simulink library "BechamoNasaOpenModels"  (R2024a)
settings: Solver=VariableStepAuto  StartTime=0.0  StopTime=10.0  RelTol=1e-3
values from neighbouring files (symbols this model uses):
  Cl_aileron_wing_1 = Cl_mat.Claileron_wing.axes1.value    [setupMavrik.m]
  Cl_aileron_wing_2 = Cl_mat.Claileron_wing.axes2.value    [setupMavrik.m]
  Cl_aileron_wing_3 = Cl_mat.Claileron_wing.axes3.value    [setupMavrik.m]
  Cl_aileron_wing_val = Cl_mat.Claileron_wing.value    [setupMavrik.m]
  Cl_elevator_tail_1 = Cl_mat.Clelevator_tail.axes1.value    [setupMavrik.m]
  Cl_elevator_tail_2 = Cl_mat.Clelevator_tail.axes2.value    [setupMavrik.m]
  Cl_elevator_tail_3 = Cl_mat.Clelevator_tail.axes3.value    [setupMavrik.m]
  Cl_elevator_tail_val = Cl_mat.Clelevator_tail.value    [setupMavrik.m]
  Cl_flap_wing_1 = Cl_mat.Clflap_wing.axes1.value    [setupMavrik.m]
  Cl_flap_wing_2 = Cl_mat.Clflap_wing.axes2.value    [setupMavrik.m]
  Cl_flap_wing_3 = Cl_mat.Clflap_wing.axes3.value    [setupMavrik.m]
  Cl_flap_wing_val = Cl_mat.Clflap_wing.value    [setupMavrik.m]
  Cl_hover_fuse_1 = Cl_mat.Clhover_fuse.axes1.value    [setupMavrik.m]
  Cl_hover_fuse_2 = Cl_mat.Clhover_fuse.axes2.value    [setupMavrik.m]
  Cl_hover_fuse_3 = Cl_mat.Clhover_fuse.axes3.value    [setupMavrik.m]
  Cl_hover_fuse_val = Cl_mat.Clhover_fuse.value    [setupMavrik.m]
  Cl_rudder_tail_1 = Cl_mat.Clrudder_tail.axes1.value    [setupMavrik.m]
  Cl_rudder_tail_2 = Cl_mat.Clrudder_tail.axes2.value    [setupMavrik.m]
  Cl_rudder_tail_3 = Cl_mat.Clrudder_tail.axes3.value    [setupMavrik.m]
  Cl_rudder_tail_val = Cl_mat.Clrudder_tail.value    [setupMavrik.m]
  Cl_tail_1 = Cl_mat.Cltail.axes1.value    [setupMavrik.m]
  Cl_tail_2 = Cl_mat.Cltail.axes2.value    [setupMavrik.m]
  Cl_tail_3 = Cl_mat.Cltail.axes3.value    [setupMavrik.m]
  Cl_tail_damp_p_1 = Cl_mat.Cltail_damp_p.axes1.value    [setupMavrik.m]
  Cl_tail_damp_p_2 = Cl_mat.Cltail_damp_p.axes2.value    [setupMavrik.m]
  Cl_tail_damp_p_3 = Cl_mat.Cltail_damp_p.axes3.value    [setupMavrik.m]
  Cl_tail_damp_p_val = Cl_mat.Cltail_damp_p.value    [setupMavrik.m]
  Cl_tail_damp_q_1 = Cl_mat.Cltail_damp_q.axes1.value    [setupMavrik.m]
  Cl_tail_damp_q_2 = Cl_mat.Cltail_damp_q.axes2.value    [setupMavrik.m]
  Cl_tail_damp_q_3 = Cl_mat.Cltail_damp_q.axes3.value    [setupMavrik.m]
  Cl_tail_damp_q_val = Cl_mat.Cltail_damp_q.value    [setupMavrik.m]
  Cl_tail_damp_r_1 = Cl_mat.Cltail_damp_r.axes1.value    [setupMavrik.m]
  Cl_tail_damp_r_2 = Cl_mat.Cltail_damp_r.axes2.value    [setupMavrik.m]
  Cl_tail_damp_r_3 = Cl_mat.Cltail_damp_r.axes3.value    [setupMavrik.m]
  Cl_tail_damp_r_val = Cl_mat.Cltail_damp_r.value    [setupMavrik.m]
  Cl_tail_val = Cl_mat.Cltail.value    [setupMavrik.m]
  Cl_wing_1 = Cl_mat.Clwing.axes1.value    [setupMavrik.m]
  Cl_wing_2 = Cl_mat.Clwing.axes2.value    [setupMavrik.m]
  Cl_wing_3 = Cl_mat.Clwing.axes3.value    [setupMavrik.m]
  Cl_wing_damp_p_1 = Cl_mat.Clwing_damp_p.axes1.value    [setupMavrik.m]
  Cl_wing_damp_p_2 = Cl_mat.Clwing_damp_p.axes2.value    [setupMavrik.m]
  Cl_wing_damp_p_3 = Cl_mat.Clwing_damp_p.axes3.value    [setupMavrik.m]
  Cl_wing_damp_p_val = Cl_mat.Clwing_damp_p.value    [setupMavrik.m]
  Cl_wing_damp_q_1 = Cl_mat.Clwing_damp_q.axes1.value    [setupMavrik.m]
  Cl_wing_damp_q_2 = Cl_mat.Clwing_damp_q.axes2.value    [setupMavrik.m]
  Cl_wing_damp_q_3 = Cl_mat.Clwing_damp_q.axes3.value    [setupMavrik.m]
  Cl_wing_damp_q_val = Cl_mat.Clwing_damp_q.value    [setupMavrik.m]
  Cl_wing_damp_r_1 = Cl_mat.Clwing_damp_r.axes1.value    [setupMavrik.m]
  Cl_wing_damp_r_2 = Cl_mat.Clwing_damp_r.axes2.value    [setupMavrik.m]
  Cl_wing_damp_r_3 = Cl_mat.Clwing_damp_r.axes3.value    [setupMavrik.m]
  Cl_wing_damp_r_val = Cl_mat.Clwing_damp_r.value    [setupMavrik.m]
  Cl_wing_val = Cl_mat.Clwing.value    [setupMavrik.m]
  Cm_aileron_wing_1 = Cm_mat.Cmaileron_wing.axes1.value    [setupMavrik.m]
  Cm_aileron_wing_2 = Cm_mat.Cmaileron_wing.axes2.value    [setupMavrik.m]
  Cm_aileron_wing_3 = Cm_mat.Cmaileron_wing.axes3.value    [setupMavrik.m]
  Cm_aileron_wing_val = Cm_mat.Cmaileron_wing.value    [setupMavrik.m]
  Cm_elevator_tail_1 = Cm_mat.Cmelevator_tail.axes1.value    [setupMavrik.m]
  Cm_elevator_tail_2 = Cm_mat.Cmelevator_tail.axes2.value    [setupMavrik.m]
  Cm_elevator_tail_3 = Cm_mat.Cmelevator_tail.axes3.value    [setupMavrik.m]
  Cm_elevator_tail_val = Cm_mat.Cmelevator_tail.value    [setupMavrik.m]
  Cm_flap_wing_1 = Cm_mat.Cmflap_wing.axes1.value    [setupMavrik.m]
  Cm_flap_wing_2 = Cm_mat.Cmflap_wing.axes2.value    [setupMavrik.m]
  Cm_flap_wing_3 = Cm_mat.Cmflap_wing.axes3.value    [setupMavrik.m]
  Cm_flap_wing_val = Cm_mat.Cmflap_wing.value    [setupMavrik.m]
  Cm_hover_fuse_1 = Cm_mat.Cmhover_fuse.axes1.value    [setupMavrik.m]
  Cm_hover_fuse_2 = Cm_mat.Cmhover_fuse.axes2.value    [setupMavrik.m]
  Cm_hover_fuse_3 = Cm_mat.Cmhover_fuse.axes3.value    [setupMavrik.m]
  Cm_hover_fuse_val = Cm_mat.Cmhover_fuse.value    [setupMavrik.m]
  Cm_rudder_tail_1 = Cm_mat.Cmrudder_tail.axes1.value    [setupMavrik.m]
  Cm_rudder_tail_2 = Cm_mat.Cmrudder_tail.axes2.value    [setupMavrik.m]
  Cm_rudder_tail_3 = Cm_mat.Cmrudder_tail.axes3.value    [setupMavrik.m]
  Cm_rudder_tail_val = Cm_mat.Cmrudder_tail.value    [setupMavrik.m]
  Cm_tail_1 = Cm_mat.Cmtail.axes1.value    [setupMavrik.m]
  Cm_tail_2 = Cm_mat.Cmtail.axes2.value    [setupMavrik.m]
  Cm_tail_3 = Cm_mat.Cmtail.axes3.value    [setupMavrik.m]
  Cm_tail_damp_p_1 = Cm_mat.Cmtail_damp_p.axes1.value    [setupMavrik.m]
  Cm_tail_damp_p_2 = Cm_mat.Cmtail_damp_p.axes2.value    [setupMavrik.m]
  Cm_tail_damp_p_3 = Cm_mat.Cmtail_damp_p.axes3.value    [setupMavrik.m]
  Cm_tail_damp_p_val = Cm_mat.Cmtail_damp_p.value    [setupMavrik.m]
  Cm_tail_damp_q_1 = Cm_mat.Cmtail_damp_q.axes1.value    [setupMavrik.m]
  Cm_tail_damp_q_2 = Cm_mat.Cmtail_damp_q.axes2.value    [setupMavrik.m]
  Cm_tail_damp_q_3 = Cm_mat.Cmtail_damp_q.axes3.value    [setupMavrik.m]
  Cm_tail_damp_q_val = Cm_mat.Cmtail_damp_q.value    [setupMavrik.m]
  Cm_tail_damp_r_1 = Cm_mat.Cmtail_damp_r.axes1.value    [setupMavrik.m]
  Cm_tail_damp_r_2 = Cm_mat.Cmtail_damp_r.axes2.value    [setupMavrik.m]
  Cm_tail_damp_r_3 = Cm_mat.Cmtail_damp_r.axes3.value    [setupMavrik.m]
  Cm_tail_damp_r_val = Cm_mat.Cmtail_damp_r.value    [setupMavrik.m]
  Cm_tail_val = Cm_mat.Cmtail.value    [setupMavrik.m]
  Cm_wing_1 = Cm_mat.Cmwing.axes1.value    [setupMavrik.m]
  Cm_wing_2 = Cm_mat.Cmwing.axes2.value    [setupMavrik.m]
  Cm_wing_3 = Cm_mat.Cmwing.axes3.value    [setupMavrik.m]
  Cm_wing_damp_p_1 = Cm_mat.Cmwing_damp_p.axes1.value    [setupMavrik.m]
  Cm_wing_damp_p_2 = Cm_mat.Cmwing_damp_p.axes2.value    [setupMavrik.m]
  Cm_wing_damp_p_3 = Cm_mat.Cmwing_damp_p.axes3.value    [setupMavrik.m]
  Cm_wing_damp_p_val = Cm_mat.Cmwing_damp_p.value    [setupMavrik.m]
  Cm_wing_damp_q_1 = Cm_mat.Cmwing_damp_q.axes1.value    [setupMavrik.m]
  Cm_wing_damp_q_2 = Cm_mat.Cmwing_damp_q.axes2.value    [setupMavrik.m]
  Cm_wing_damp_q_3 = Cm_mat.Cmwing_damp_q.axes3.value    [setupMavrik.m]
  Cm_wing_damp_q_val = Cm_mat.Cmwing_damp_q.value    [setupMavrik.m]
  Cm_wing_damp_r_1 = Cm_mat.Cmwing_damp_r.axes1.value    [setupMavrik.m]
  Cm_wing_damp_r_2 = Cm_mat.Cmwing_damp_r.axes2.value    [setupMavrik.m]
  Cm_wing_damp_r_3 = Cm_mat.Cmwing_damp_r.axes3.value    [setupMavrik.m]
  Cm_wing_damp_r_val = Cm_mat.Cmwing_damp_r.value    [setupMavrik.m]
  Cm_wing_val = Cm_mat.Cmwing.value    [setupMavrik.m]
  Cn_aileron_wing_1 = Cn_mat.Cnaileron_wing.axes1.value    [setupMavrik.m]
  Cn_aileron_wing_2 = Cn_mat.Cnaileron_wing.axes2.value    [setupMavrik.m]
  Cn_aileron_wing_3 = Cn_mat.Cnaileron_wing.axes3.value    [setupMavrik.m]
  Cn_aileron_wing_val = Cn_mat.Cnaileron_wing.value    [setupMavrik.m]
  Cn_elevator_tail_1 = Cn_mat.Cnelevator_tail.axes1.value    [setupMavrik.m]
  Cn_elevator_tail_2 = Cn_mat.Cnelevator_tail.axes2.value    [setupMavrik.m]
  Cn_elevator_tail_3 = Cn_mat.Cnelevator_tail.axes3.value    [setupMavrik.m]
  Cn_elevator_tail_val = Cn_mat.Cnelevator_tail.value    [setupMavrik.m]
  Cn_flap_wing_1 = Cn_mat.Cnflap_wing.axes1.value    [setupMavrik.m]
  Cn_flap_wing_2 = Cn_mat.Cnflap_wing.axes2.value    [setupMavrik.m]
  Cn_flap_wing_3 = Cn_mat.Cnflap_wing.axes3.value    [setupMavrik.m]
  Cn_flap_wing_val = Cn_mat.Cnflap_wing.value    [setupMavrik.m]
  Cn_hover_fuse_1 = Cn_mat.Cnhover_fuse.axes1.value    [setupMavrik.m]
  Cn_hover_fuse_2 = Cn_mat.Cnhover_fuse.axes2.value    [setupMavrik.m]
  Cn_hover_fuse_3 = Cn_mat.Cnhover_fuse.axes3.value    [setupMavrik.m]
  Cn_hover_fuse_val = Cn_mat.Cnhover_fuse.value    [setupMavrik.m]
  ... (+318 more)
libraries: matrix_library x15, shared6dof x1, sharedtransform x1
(part 5 of 19)

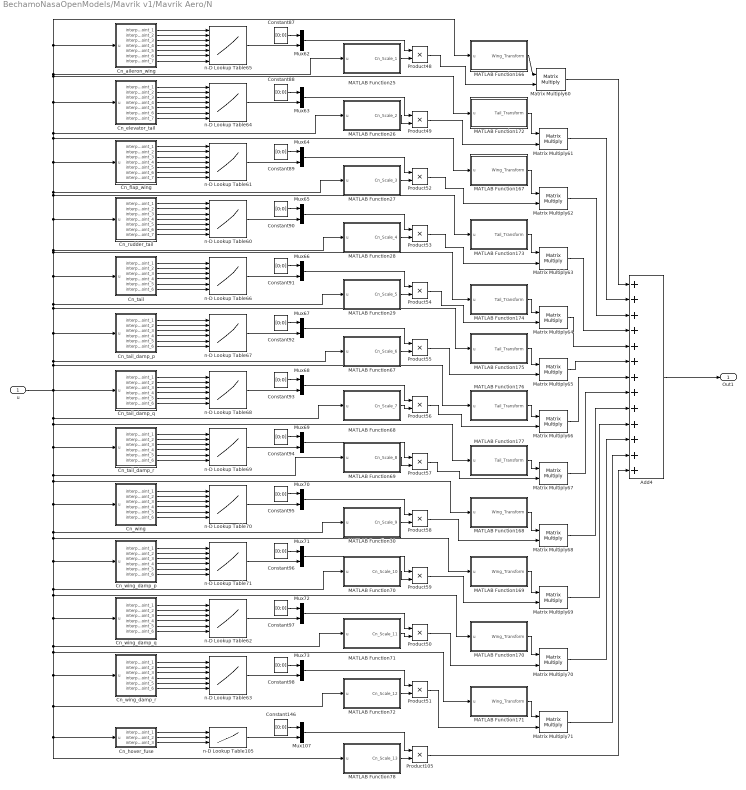
== system BechamoNasaOpenModels/Mavrik v1/Mavrik Aero/N ==
  u : Inport
  Add4 : Sum  Inputs=+++++++++++++
  Cn_aileron_wing : MATLAB Function  TreatAsAtomicUnit=on
  Cn_elevator_tail : MATLAB Function  TreatAsAtomicUnit=on
  Cn_flap_wing : MATLAB Function  TreatAsAtomicUnit=on
  Cn_hover_fuse : MATLAB Function  TreatAsAtomicUnit=on
  Cn_rudder_tail : MATLAB Function  TreatAsAtomicUnit=on
  Cn_tail : MATLAB Function  TreatAsAtomicUnit=on
  Cn_tail_damp_p : MATLAB Function  TreatAsAtomicUnit=on
  Cn_tail_damp_q : MATLAB Function  TreatAsAtomicUnit=on
  Cn_tail_damp_r : MATLAB Function  TreatAsAtomicUnit=on
  Cn_wing : MATLAB Function  TreatAsAtomicUnit=on
  Cn_wing_damp_p : MATLAB Function  TreatAsAtomicUnit=on
  Cn_wing_damp_q : MATLAB Function  TreatAsAtomicUnit=on
  Cn_wing_damp_r : MATLAB Function  TreatAsAtomicUnit=on
  Constant{87..98,146} (13 alike) : Constant  Value=[0;0]
  MATLAB Function166 : MATLAB Function  TreatAsAtomicUnit=on
  MATLAB Function167 : MATLAB Function  TreatAsAtomicUnit=on
  MATLAB Function168 : MATLAB Function  TreatAsAtomicUnit=on
  MATLAB Function169 : MATLAB Function  TreatAsAtomicUnit=on
  MATLAB Function170 : MATLAB Function  TreatAsAtomicUnit=on
  MATLAB Function171 : MATLAB Function  TreatAsAtomicUnit=on
  MATLAB Function172 : MATLAB Function  TreatAsAtomicUnit=on
  MATLAB Function173 : MATLAB Function  TreatAsAtomicUnit=on
  MATLAB Function174 : MATLAB Function  TreatAsAtomicUnit=on
  MATLAB Function175 : MATLAB Function  TreatAsAtomicUnit=on
  MATLAB Function176 : MATLAB Function  TreatAsAtomicUnit=on
  MATLAB Function177 : MATLAB Function  TreatAsAtomicUnit=on
  MATLAB Function25 : MATLAB Function  TreatAsAtomicUnit=on
  MATLAB Function26 : MATLAB Function  TreatAsAtomicUnit=on
  MATLAB Function27 : MATLAB Function  TreatAsAtomicUnit=on
  MATLAB Function28 : MATLAB Function  TreatAsAtomicUnit=on
  MATLAB Function29 : MATLAB Function  TreatAsAtomicUnit=on
  MATLAB Function30 : MATLAB Function  TreatAsAtomicUnit=on
  MATLAB Function67 : MATLAB Function  TreatAsAtomicUnit=on
  MATLAB Function68 : MATLAB Function  TreatAsAtomicUnit=on
  MATLAB Function69 : MATLAB Function  TreatAsAtomicUnit=on
  MATLAB Function70 : MATLAB Function  TreatAsAtomicUnit=on
  MATLAB Function71 : MATLAB Function  TreatAsAtomicUnit=on
  MATLAB Function72 : MATLAB Function  TreatAsAtomicUnit=on
  MATLAB Function78 : MATLAB Function  TreatAsAtomicUnit=on
  Matrix Multiply{60..71} (12 alike) : Product  Multiplication=Matrix(*)
  Mux{62..73,107} (13 alike) : Mux  Inputs=2
  Product{48..59,105} (13 alike) : Product
  n-D Lookup Table105 : Lookup_n-D  NumberOfTableDimensions=3  BreakpointsForDimension1=Cn_hover_fuse_1  BreakpointsForDimension2=Cn_hover_fuse_2  BreakpointsForDimension3=Cn_hover_fuse_3  BreakpointsForDimension4=CX_wing_damp_r_4  BreakpointsForDimension5=CX_wing_damp_r_5  BreakpointsForDimension6=CX_wing_damp_r_6  BreakpointsForDimension7=CX_flap_wing_7  Table=Cn_hover_fuse_val  InternalRulePriority=Speed  OutDataTypeStr=Inherit: Inherit via back propagation  RndMeth=Simplest
      settings: InputPortMap=u0,u1,u2
  n-D Lookup Table60 : Lookup_n-D  NumberOfTableDimensions=7  BreakpointsForDimension1=Cn_rudder_tail_1  BreakpointsForDimension2=Cn_rudder_tail_2  BreakpointsForDimension3=Cn_rudder_tail_3  BreakpointsForDimension4=Cn_rudder_tail_4  BreakpointsForDimension5=Cn_rudder_tail_5  BreakpointsForDimension6=Cn_rudder_tail_6  BreakpointsForDimension7=Cn_rudder_tail_7  Table=Cn_rudder_tail_val  InternalRulePriority=Speed  OutDataTypeStr=Inherit: Inherit via back propagation  RndMeth=Simplest
      settings: InputPortMap=u0,u1,u2,u3,u4,u5,u6
  n-D Lookup Table61 : Lookup_n-D  NumberOfTableDimensions=7  BreakpointsForDimension1=Cn_flap_wing_1  BreakpointsForDimension2=Cn_flap_wing_2  BreakpointsForDimension3=Cn_flap_wing_3  BreakpointsForDimension4=Cn_flap_wing_4  BreakpointsForDimension5=Cn_flap_wing_5  BreakpointsForDimension6=Cn_flap_wing_6  BreakpointsForDimension7=Cn_flap_wing_7  Table=Cn_flap_wing_val  InternalRulePriority=Speed  OutDataTypeStr=Inherit: Inherit via back propagation  RndMeth=Simplest
      settings: InputPortMap=u0,u1,u2,u3,u4,u5,u6
  n-D Lookup Table62 : Lookup_n-D  NumberOfTableDimensions=6  BreakpointsForDimension1=Cn_wing_damp_q_1  BreakpointsForDimension2=Cn_wing_damp_q_2  BreakpointsForDimension3=Cn_wing_damp_q_3  BreakpointsForDimension4=Cn_wing_damp_q_4  BreakpointsForDimension5=Cn_wing_damp_q_5  BreakpointsForDimension6=Cn_wing_damp_q_6  BreakpointsForDimension7=CX_flap_wing_7  Table=Cn_wing_damp_q_val  InternalRulePriority=Speed  OutDataTypeStr=Inherit: Inherit via back propagation  RndMeth=Simplest
      settings: InputPortMap=u0,u1,u2,u3,u4,u5
  n-D Lookup Table63 : Lookup_n-D  NumberOfTableDimensions=6  BreakpointsForDimension1=Cn_wing_damp_r_1  BreakpointsForDimension2=Cn_wing_damp_r_2  BreakpointsForDimension3=Cn_wing_damp_r_3  BreakpointsForDimension4=Cn_wing_damp_r_4  BreakpointsForDimension5=Cn_wing_damp_r_5  BreakpointsForDimension6=Cn_wing_damp_r_6  BreakpointsForDimension7=CX_flap_wing_7  Table=Cn_wing_damp_r_val  InternalRulePriority=Speed  OutDataTypeStr=Inherit: Inherit via back propagation  RndMeth=Simplest
      settings: InputPortMap=u0,u1,u2,u3,u4,u5
  n-D Lookup Table64 : Lookup_n-D  NumberOfTableDimensions=7  BreakpointsForDimension1=Cn_elevator_tail_1  BreakpointsForDimension2=Cn_elevator_tail_2  BreakpointsForDimension3=Cn_elevator_tail_3  BreakpointsForDimension4=Cn_elevator_tail_4  BreakpointsForDimension5=Cn_elevator_tail_5  BreakpointsForDimension6=Cn_elevator_tail_6  BreakpointsForDimension7=Cn_elevator_tail_7  Table=Cn_elevator_tail_val  InternalRulePriority=Speed  OutDataTypeStr=Inherit: Inherit via back propagation  RndMeth=Simplest
      settings: InputPortMap=u0,u1,u2,u3,u4,u5,u6
  n-D Lookup Table65 : Lookup_n-D  NumberOfTableDimensions=7  BreakpointsForDimension1=Cn_aileron_wing_1  BreakpointsForDimension2=Cn_aileron_wing_2  BreakpointsForDimension3=Cn_aileron_wing_3  BreakpointsForDimension4=Cn_aileron_wing_4  BreakpointsForDimension5=Cn_aileron_wing_5  BreakpointsForDimension6=Cn_aileron_wing_6  BreakpointsForDimension7=Cn_aileron_wing_7  Table=Cn_aileron_wing_val  InternalRulePriority=Speed  OutDataTypeStr=Inherit: Inherit via back propagation  RndMeth=Simplest
      settings: InputPortMap=u0,u1,u2,u3,u4,u5,u6
  n-D Lookup Table66 : Lookup_n-D  NumberOfTableDimensions=6  BreakpointsForDimension1=Cn_tail_1  BreakpointsForDimension2=Cn_tail_2  BreakpointsForDimension3=Cn_tail_3  BreakpointsForDimension4=Cn_tail_4  BreakpointsForDimension5=Cn_tail_5  BreakpointsForDimension6=Cn_tail_6  BreakpointsForDimension7=CX_tail_7  Table=Cn_tail_val  InternalRulePriority=Speed  OutDataTypeStr=Inherit: Inherit via back propagation  RndMeth=Simplest
      settings: InputPortMap=u0,u1,u2,u3,u4,u5
  n-D Lookup Table67 : Lookup_n-D  NumberOfTableDimensions=6  BreakpointsForDimension1=Cn_tail_damp_p_1  BreakpointsForDimension2=Cn_tail_damp_p_2  BreakpointsForDimension3=Cn_tail_damp_p_3  BreakpointsForDimension4=Cn_tail_damp_p_4  BreakpointsForDimension5=Cn_tail_damp_p_5  BreakpointsForDimension6=Cn_tail_damp_p_6  BreakpointsForDimension7=CX_tail_7  Table=Cn_tail_damp_p_val  InternalRulePriority=Speed  OutDataTypeStr=Inherit: Inherit via back propagation  RndMeth=Simplest
      settings: InputPortMap=u0,u1,u2,u3,u4,u5
  n-D Lookup Table68 : Lookup_n-D  NumberOfTableDimensions=6  BreakpointsForDimension1=Cn_tail_damp_q_1  BreakpointsForDimension2=Cn_tail_damp_q_2  BreakpointsForDimension3=Cn_tail_damp_q_3  BreakpointsForDimension4=Cn_tail_damp_q_4  BreakpointsForDimension5=Cn_tail_damp_q_5  BreakpointsForDimension6=Cn_tail_damp_q_6  BreakpointsForDimension7=CX_tail_7  Table=Cn_tail_damp_q_val  InternalRulePriority=Speed  OutDataTypeStr=Inherit: Inherit via back propagation  RndMeth=Simplest
      settings: InputPortMap=u0,u1,u2,u3,u4,u5
  n-D Lookup Table69 : Lookup_n-D  NumberOfTableDimensions=6  BreakpointsForDimension1=Cn_tail_damp_r_1  BreakpointsForDimension2=Cn_tail_damp_r_2  BreakpointsForDimension3=Cn_tail_damp_r_3  BreakpointsForDimension4=Cn_tail_damp_r_4  BreakpointsForDimension5=Cn_tail_damp_r_5  BreakpointsForDimension6=Cn_tail_damp_r_6  BreakpointsForDimension7=CX_tail_7  Table=Cn_tail_damp_r_val  InternalRulePriority=Speed  OutDataTypeStr=Inherit: Inherit via back propagation  RndMeth=Simplest
      settings: InputPortMap=u0,u1,u2,u3,u4,u5
  n-D Lookup Table70 : Lookup_n-D  NumberOfTableDimensions=6  BreakpointsForDimension1=Cn_wing_1  BreakpointsForDimension2=Cn_wing_2  BreakpointsForDimension3=Cn_wing_3  BreakpointsForDimension4=Cn_wing_4  BreakpointsForDimension5=Cn_wing_5  BreakpointsForDimension6=Cn_wing_6  BreakpointsForDimension7=CX_flap_wing_7  Table=Cn_wing_val  InternalRulePriority=Speed  OutDataTypeStr=Inherit: Inherit via back propagation  RndMeth=Simplest
      settings: InputPortMap=u0,u1,u2,u3,u4,u5
  n-D Lookup Table71 : Lookup_n-D  NumberOfTableDimensions=6  BreakpointsForDimension1=Cn_wing_damp_p_1  BreakpointsForDimension2=Cn_wing_damp_p_2  BreakpointsForDimension3=Cn_wing_damp_p_3  BreakpointsForDimension4=Cn_wing_damp_p_4  BreakpointsForDimension5=Cn_wing_damp_p_5  BreakpointsForDimension6=Cn_wing_damp_p_6  BreakpointsForDimension7=CX_flap_wing_7  Table=Cn_wing_damp_p_val  InternalRulePriority=Speed  OutDataTypeStr=Inherit: Inherit via back propagation  RndMeth=Simplest
      settings: InputPortMap=u0,u1,u2,u3,u4,u5
  Out1 : Outport
  wires:
  Cn_tail_damp_p/4(interp_point_4) -> n-D Lookup Table67/4
  Mux65/1 -> Product53/1
  n-D Lookup Table68/1 -> Mux68/2
  Product57/1 -> Matrix Multiply67/2
  n-D Lookup Table63/1 -> Mux73/2
  Constant96/1 -> Mux71/1
  n-D Lookup Table71/1 -> Mux71/2
  Matrix Multiply68/1 -> Add4/9
  Product54/1 -> Matrix Multiply64/2
  Matrix Multiply60/1 -> Add4/1
  Cn_flap_wing/7(interp_point_7) -> n-D Lookup Table61/7
  Cn_tail_damp_q/4(interp_point_4) -> n-D Lookup Table68/4
  Constant94/1 -> Mux69/1
  Cn_wing_damp_r/4(interp_point_4) -> n-D Lookup Table63/4
  Matrix Multiply61/1 -> Add4/2
  Cn_tail_damp_q/3(interp_point_3) -> n-D Lookup Table68/3
  Cn_tail_damp_p/5(interp_point_5) -> n-D Lookup Table67/5
  Mux62/1 -> Product48/1
  Cn_wing_damp_p/6(interp_point_6) -> n-D Lookup Table71/6
  Product48/1 -> Matrix Multiply60/2
  Mux66/1 -> Product54/1
  Cn_rudder_tail/7(interp_point_7) -> n-D Lookup Table60/7
  Cn_elevator_tail/5(interp_point_5) -> n-D Lookup Table64/5
  Constant92/1 -> Mux67/1
  Product52/1 -> Matrix Multiply62/2
  Cn_wing/1(interp_point_1) -> n-D Lookup Table70/1
  Cn_flap_wing/1(interp_point_1) -> n-D Lookup Table61/1
  Product50/1 -> Matrix Multiply70/2
  Matrix Multiply66/1 -> Add4/7
  Mux72/1 -> Product50/1
  Mux63/1 -> Product49/1
  n-D Lookup Table60/1 -> Mux65/2
  Mux71/1 -> Product59/1
  Mux68/1 -> Product56/1
  n-D Lookup Table65/1 -> Mux62/2
  Cn_tail/1(interp_point_1) -> n-D Lookup Table66/1
  Matrix Multiply70/1 -> Add4/11
  Cn_tail/4(interp_point_4) -> n-D Lookup Table66/4
  Mux64/1 -> Product52/1
  Matrix Multiply63/1 -> Add4/4
  MATLAB Function30/1(Cn_Scale_9) -> Product58/2
  Cn_aileron_wing/4(interp_point_4) -> n-D Lookup Table65/4
  Mux69/1 -> Product57/1
  n-D Lookup Table64/1 -> Mux63/2
  Cn_wing/6(interp_point_6) -> n-D Lookup Table70/6
  Constant88/1 -> Mux63/1
  Matrix Multiply67/1 -> Add4/8
  Product56/1 -> Matrix Multiply66/2
  Cn_tail_damp_p/6(interp_point_6) -> n-D Lookup Table67/6
  Constant91/1 -> Mux66/1
  MATLAB Function70/1(Cn_Scale_10) -> Product59/2
  Constant89/1 -> Mux64/1
  Cn_tail_damp_p/2(interp_point_2) -> n-D Lookup Table67/2
  Constant95/1 -> Mux70/1
  Cn_aileron_wing/2(interp_point_2) -> n-D Lookup Table65/2
  MATLAB Function26/1(Cn_Scale_2) -> Product49/2
  Cn_tail_damp_r/4(interp_point_4) -> n-D Lookup Table69/4
  MATLAB Function173/1(Tail_Transform) -> Matrix Multiply63/1
  Matrix Multiply69/1 -> Add4/10
  Cn_flap_wing/3(interp_point_3) -> n-D Lookup Table61/3
  MATLAB Function28/1(Cn_Scale_4) -> Product53/2
  MATLAB Function67/1(Cn_Scale_6) -> Product55/2
  Cn_tail_damp_q/2(interp_point_2) -> n-D Lookup Table68/2
  Cn_wing/5(interp_point_5) -> n-D Lookup Table70/5
  Product59/1 -> Matrix Multiply69/2
  Constant90/1 -> Mux65/1
  Cn_tail_damp_p/1(interp_point_1) -> n-D Lookup Table67/1
  MATLAB Function69/1(Cn_Scale_8) -> Product57/2
  MATLAB Function171/1(Wing_Transform) -> Matrix Multiply71/1
  Cn_elevator_tail/3(interp_point_3) -> n-D Lookup Table64/3
  Cn_hover_fuse/3(interp_point_3) -> n-D Lookup Table105/3
  Cn_flap_wing/6(interp_point_6) -> n-D Lookup Table61/6
  Cn_tail/2(interp_point_2) -> n-D Lookup Table66/2
  Cn_wing/4(interp_point_4) -> n-D Lookup Table70/4
  Product55/1 -> Matrix Multiply65/2
  Mux73/1 -> Product51/1
  Cn_hover_fuse/1(interp_point_1) -> n-D Lookup Table105/1
  Product105/1 -> Add4/13
  Mux107/1 -> Product105/1
  Cn_elevator_tail/1(interp_point_1) -> n-D Lookup Table64/1
  Cn_wing_damp_q/4(interp_point_4) -> n-D Lookup Table62/4
  Matrix Multiply62/1 -> Add4/3
  n-D Lookup Table61/1 -> Mux64/2
  Constant87/1 -> Mux62/1
  Constant97/1 -> Mux72/1
  Cn_wing_damp_p/4(interp_point_4) -> n-D Lookup Table71/4
  n-D Lookup Table69/1 -> Mux69/2
  Constant146/1 -> Mux107/1
  Cn_elevator_tail/4(interp_point_4) -> n-D Lookup Table64/4
  Product49/1 -> Matrix Multiply61/2
  Cn_wing_damp_r/6(interp_point_6) -> n-D Lookup Table63/6
  Cn_aileron_wing/5(interp_point_5) -> n-D Lookup Table65/5
  Product53/1 -> Matrix Multiply63/2
  Cn_aileron_wing/7(interp_point_7) -> n-D Lookup Table65/7
  Cn_tail/6(interp_point_6) -> n-D Lookup Table66/6
  MATLAB Function27/1(Cn_Scale_3) -> Product52/2
  MATLAB Function176/1(Tail_Transform) -> Matrix Multiply66/1
  MATLAB Function167/1(Wing_Transform) -> Matrix Multiply62/1
  Cn_rudder_tail/3(interp_point_3) -> n-D Lookup Table60/3
  Matrix Multiply71/1 -> Add4/12
  Cn_tail_damp_r/2(interp_point_2) -> n-D Lookup Table69/2
  Cn_tail/5(interp_point_5) -> n-D Lookup Table66/5
  Matrix Multiply64/1 -> Add4/5
  Cn_tail_damp_q/1(interp_point_1) -> n-D Lookup Table68/1
  Cn_tail_damp_p/3(interp_point_3) -> n-D Lookup Table67/3
  Cn_flap_wing/2(interp_point_2) -> n-D Lookup Table61/2
  Cn_wing_damp_q/6(interp_point_6) -> n-D Lookup Table62/6
  MATLAB Function25/1(Cn_Scale_1) -> Product48/2
  n-D Lookup Table70/1 -> Mux70/2
  Cn_rudder_tail/1(interp_point_1) -> n-D Lookup Table60/1
  Cn_tail_damp_q/5(interp_point_5) -> n-D Lookup Table68/5
  Constant93/1 -> Mux68/1
  n-D Lookup Table67/1 -> Mux67/2
  MATLAB Function175/1(Tail_Transform) -> Matrix Multiply65/1
  Cn_flap_wing/5(interp_point_5) -> n-D Lookup Table61/5
  Cn_flap_wing/4(interp_point_4) -> n-D Lookup Table61/4
  Cn_rudder_tail/5(interp_point_5) -> n-D Lookup Table60/5
  Cn_wing_damp_p/3(interp_point_3) -> n-D Lookup Table71/3
  Cn_elevator_tail/2(interp_point_2) -> n-D Lookup Table64/2
  Cn_tail_damp_q/6(interp_point_6) -> n-D Lookup Table68/6
  Cn_rudder_tail/4(interp_point_4) -> n-D Lookup Table60/4
  Cn_aileron_wing/6(interp_point_6) -> n-D Lookup Table65/6
  Cn_wing_damp_r/3(interp_point_3) -> n-D Lookup Table63/3
  MATLAB Function172/1(Tail_Transform) -> Matrix Multiply61/1
  Cn_wing_damp_r/5(interp_point_5) -> n-D Lookup Table63/5
  Cn_elevator_tail/7(interp_point_7) -> n-D Lookup Table64/7
  Cn_tail_damp_r/3(interp_point_3) -> n-D Lookup Table69/3
  Cn_tail_damp_r/6(interp_point_6) -> n-D Lookup Table69/6
  Cn_aileron_wing/1(interp_point_1) -> n-D Lookup Table65/1
  Cn_tail/3(interp_point_3) -> n-D Lookup Table66/3
  Cn_wing_damp_p/5(interp_point_5) -> n-D Lookup Table71/5
  Cn_wing_damp_p/2(interp_point_2) -> n-D Lookup Table71/2
  Cn_wing_damp_q/2(interp_point_2) -> n-D Lookup Table62/2
  Cn_wing_damp_r/2(interp_point_2) -> n-D Lookup Table63/2
  Cn_tail_damp_r/5(interp_point_5) -> n-D Lookup Table69/5
  Cn_wing/3(interp_point_3) -> n-D Lookup Table70/3
  MATLAB Function166/1(Wing_Transform) -> Matrix Multiply60/1
  Product51/1 -> Matrix Multiply71/2
  Cn_wing_damp_q/3(interp_point_3) -> n-D Lookup Table62/3
  n-D Lookup Table62/1 -> Mux72/2
  Add4/1 -> Out1/1
  Mux70/1 -> Product58/1
  Cn_wing_damp_q/5(interp_point_5) -> n-D Lookup Table62/5
  Mux67/1 -> Product55/1
  MATLAB Function168/1(Wing_Transform) -> Matrix Multiply68/1
  n-D Lookup Table66/1 -> Mux66/2
  Matrix Multiply65/1 -> Add4/6
  Constant98/1 -> Mux73/1
  MATLAB Function170/1(Wing_Transform) -> Matrix Multiply70/1
  MATLAB Function177/1(Tail_Transform) -> Matrix Multiply67/1
  MATLAB Function169/1(Wing_Transform) -> Matrix Multiply69/1
  Cn_elevator_tail/6(interp_point_6) -> n-D Lookup Table64/6
  MATLAB Function29/1(Cn_Scale_5) -> Product54/2
  Cn_aileron_wing/3(interp_point_3) -> n-D Lookup Table65/3
  MATLAB Function78/1(Cn_Scale_13) -> Product105/2
  Cn_wing/2(interp_point_2) -> n-D Lookup Table70/2
  Product58/1 -> Matrix Multiply68/2
  MATLAB Function68/1(Cn_Scale_7) -> Product56/2
  Cn_wing_damp_p/1(interp_point_1) -> n-D Lookup Table71/1
  MATLAB Function71/1(Cn_Scale_11) -> Product50/2
  Cn_wing_damp_q/1(interp_point_1) -> n-D Lookup Table62/1
  n-D Lookup Table105/1 -> Mux107/2
  Cn_rudder_tail/2(interp_point_2) -> n-D Lookup Table60/2
  Cn_wing_damp_r/1(interp_point_1) -> n-D Lookup Table63/1
  Cn_hover_fuse/2(interp_point_2) -> n-D Lookup Table105/2
  MATLAB Function174/1(Tail_Transform) -> Matrix Multiply64/1
  Cn_rudder_tail/6(interp_point_6) -> n-D Lookup Table60/6
  Cn_tail_damp_r/1(interp_point_1) -> n-D Lookup Table69/1
  MATLAB Function72/1(Cn_Scale_12) -> Product51/2
  u/1 -> MATLAB Function68/1(u), MATLAB Function69/1(u), MATLAB Function168/1(u), Cn_wing/1(u), MATLAB Function30/1(u), MATLAB Function169/1(u), Cn_wing_damp_p/1(u), MATLAB Function70/1(u), MATLAB Function170/1(u), Cn_wing_damp_q/1(u), MATLAB Function71/1(u), MATLAB Function171/1(u), Cn_wing_damp_r/1(u), MATLAB Function72/1(u), Cn_hover_fuse/1(u), MATLAB Function78/1(u), Cn_tail_damp_r/1(u), MATLAB Function177/1(u), MATLAB Function176/1(u), MATLAB Function67/1(u), Cn_tail_damp_p/1(u), MATLAB Function175/1(u), MATLAB Function29/1(u), Cn_tail/1(u), MATLAB Function174/1(u), MATLAB Function28/1(u), Cn_rudder_tail/1(u), MATLAB Function173/1(u), Cn_flap_wing/1(u), MATLAB Function167/1(u), MATLAB Function26/1(u), Cn_elevator_tail/1(u), Cn_aileron_wing/1(u), MATLAB Function166/1(u), MATLAB Function25/1(u), MATLAB Function172/1(u), MATLAB Function27/1(u), Cn_tail_damp_q/1(u)

== matlab function BechamoNasaOpenModels/Mavrik v1/Mavrik Aero/Ct/Ct_right_9 ==
  data: u input size=[1 45]; interp_point_1 output; interp_point_2 output; interp_point_3 output; interp_point_4 output
function [interp_point_1, interp_point_2, interp_point_3, interp_point_4] = fcn(u)

% Find Interpolation Points
variable_indices = struct('U', 1, 'alpha', 2, 'beta', 3, 'p', 4, 'q', 5, 'r', 6, 'wing_alpha', 7, 'wing_beta', 8, 'wing_RPM', 9, 'left_alpha', 10,...
    'right_alpha', 11, 'left_beta', 12, 'right_beta', 13, 'wing_prop_alpha', 14, 'wing_prop_beta', 15, 'tail_alpha', 16, 'tail_beta', 17, 'tail_RPM', 18, 'tailLeft_alpha', 19, 'tailRight_alpha', 20,...
    'tailLeft_beta', 21, 'tailRight_beta', 22, 'tail_prop_alpha', 23, 'tail_prop_beta', 24, 'Q', 25, 'aileron', 26, 'elevator', 27, 'flap', 28, 'rudder', 29, 'wing_tilt', 30,...
    'tail_tilt', 31, 'RPM_tailLeft', 32, 'RPM_tailRight', 33, 'RPM_leftOut1', 34, 'RPM_left2', 35, 'RPM_left3', 36, 'RPM_left4', 37, 'RPM_left5', 38, 'RPM_left6In', 39, 'RPM_right7In', 40,...
    'RPM_right8', 41, 'RPM_right9', 42, 'RPM_right10', 43, 'RPM_right11', 44, 'RPM_right12Out', 45);

interp_point_1  = u(variable_indices.U);
interp_point_2  = u(variable_indices.wing_RPM);
interp_point_3  = u(variable_indices.wing_prop_alpha);
interp_point_4  = u(variable_indices.wing_prop_beta);

end

% y = [U, alpha, beta, p, q, r, wing_alpha, wing_beta, wing_RPM, left_alpha, right_alpha, left_beta, right_beta, wing_prop_alpha, wing_prop_beta, ...
    % tail_alpha, tail_beta, tail_RPM, tailLeft_alpha, tailRight_alpha, tailLeft_beta, tailRight_beta, tail_prop_alpha, ...
    % tail_prop_beta, Q, aileron, elevator, flap, rudder, wing_tilt, tail_tilt, RPM_tailLeft, RPM_tailRight, RPM_leftOut1, RPM_left2, ...
    % RPM_left3, RPM_left4, RPM_left5, RPM_left6In, RPM_right7In, RPM_right8, RPM_right9, RPM_right10, RPM_right11, RPM_right12Out];

== matlab function BechamoNasaOpenModels/Mavrik v1/Mavrik Aero/Ct/Ct_right_10 ==
  data: u input size=[1 45]; interp_point_1 output; interp_point_2 output; interp_point_3 output; interp_point_4 output
function [interp_point_1, interp_point_2, interp_point_3, interp_point_4] = fcn(u)

% Find Interpolation Points
variable_indices = struct('U', 1, 'alpha', 2, 'beta', 3, 'p', 4, 'q', 5, 'r', 6, 'wing_alpha', 7, 'wing_beta', 8, 'wing_RPM', 9, 'left_alpha', 10,...
    'right_alpha', 11, 'left_beta', 12, 'right_beta', 13, 'wing_prop_alpha', 14, 'wing_prop_beta', 15, 'tail_alpha', 16, 'tail_beta', 17, 'tail_RPM', 18, 'tailLeft_alpha', 19, 'tailRight_alpha', 20,...
    'tailLeft_beta', 21, 'tailRight_beta', 22, 'tail_prop_alpha', 23, 'tail_prop_beta', 24, 'Q', 25, 'aileron', 26, 'elevator', 27, 'flap', 28, 'rudder', 29, 'wing_tilt', 30,...
    'tail_tilt', 31, 'RPM_tailLeft', 32, 'RPM_tailRight', 33, 'RPM_leftOut1', 34, 'RPM_left2', 35, 'RPM_left3', 36, 'RPM_left4', 37, 'RPM_left5', 38, 'RPM_left6In', 39, 'RPM_right7In', 40,...
    'RPM_right8', 41, 'RPM_right9', 42, 'RPM_right10', 43, 'RPM_right11', 44, 'RPM_right12Out', 45);

interp_point_1  = u(variable_indices.U);
interp_point_2  = u(variable_indices.wing_RPM);
interp_point_3  = u(variable_indices.wing_prop_alpha);
interp_point_4  = u(variable_indices.wing_prop_beta);

end

% y = [U, alpha, beta, p, q, r, wing_alpha, wing_beta, wing_RPM, left_alpha, right_alpha, left_beta, right_beta, wing_prop_alpha, wing_prop_beta, ...
    % tail_alpha, tail_beta, tail_RPM, tailLeft_alpha, tailRight_alpha, tailLeft_beta, tailRight_beta, tail_prop_alpha, ...
    % tail_prop_beta, Q, aileron, elevator, flap, rudder, wing_tilt, tail_tilt, RPM_tailLeft, RPM_tailRight, RPM_leftOut1, RPM_left2, ...
    % RPM_left3, RPM_left4, RPM_left5, RPM_left6In, RPM_right7In, RPM_right8, RPM_right9, RPM_right10, RPM_right11, RPM_right12Out];

== matlab function BechamoNasaOpenModels/Mavrik v1/Mavrik Aero/Ct/Ct_right_11 ==
  data: u input size=[1 45]; interp_point_1 output; interp_point_2 output; interp_point_3 output; interp_point_4 output
function [interp_point_1, interp_point_2, interp_point_3, interp_point_4] = fcn(u)

% Find Interpolation Points
variable_indices = struct('U', 1, 'alpha', 2, 'beta', 3, 'p', 4, 'q', 5, 'r', 6, 'wing_alpha', 7, 'wing_beta', 8, 'wing_RPM', 9, 'left_alpha', 10,...
    'right_alpha', 11, 'left_beta', 12, 'right_beta', 13, 'wing_prop_alpha', 14, 'wing_prop_beta', 15, 'tail_alpha', 16, 'tail_beta', 17, 'tail_RPM', 18, 'tailLeft_alpha', 19, 'tailRight_alpha', 20,...
    'tailLeft_beta', 21, 'tailRight_beta', 22, 'tail_prop_alpha', 23, 'tail_prop_beta', 24, 'Q', 25, 'aileron', 26, 'elevator', 27, 'flap', 28, 'rudder', 29, 'wing_tilt', 30,...
    'tail_tilt', 31, 'RPM_tailLeft', 32, 'RPM_tailRight', 33, 'RPM_leftOut1', 34, 'RPM_left2', 35, 'RPM_left3', 36, 'RPM_left4', 37, 'RPM_left5', 38, 'RPM_left6In', 39, 'RPM_right7In', 40,...
    'RPM_right8', 41, 'RPM_right9', 42, 'RPM_right10', 43, 'RPM_right11', 44, 'RPM_right12Out', 45);

interp_point_1  = u(variable_indices.U);
interp_point_2  = u(variable_indices.wing_RPM);
interp_point_3  = u(variable_indices.wing_prop_alpha);
interp_point_4  = u(variable_indices.wing_prop_beta);

end

% y = [U, alpha, beta, p, q, r, wing_alpha, wing_beta, wing_RPM, left_alpha, right_alpha, left_beta, right_beta, wing_prop_alpha, wing_prop_beta, ...
    % tail_alpha, tail_beta, tail_RPM, tailLeft_alpha, tailRight_alpha, tailLeft_beta, tailRight_beta, tail_prop_alpha, ...
    % tail_prop_beta, Q, aileron, elevator, flap, rudder, wing_tilt, tail_tilt, RPM_tailLeft, RPM_tailRight, RPM_leftOut1, RPM_left2, ...
    % RPM_left3, RPM_left4, RPM_left5, RPM_left6In, RPM_right7In, RPM_right8, RPM_right9, RPM_right10, RPM_right11, RPM_right12Out];

== matlab function BechamoNasaOpenModels/Mavrik v1/Mavrik Aero/Ct/Ct_right_12_out ==
  data: u input size=[1 45]; interp_point_1 output; interp_point_2 output; interp_point_3 output; interp_point_4 output
function [interp_point_1, interp_point_2, interp_point_3, interp_point_4] = fcn(u)

% Find Interpolation Points
variable_indices = struct('U', 1, 'alpha', 2, 'beta', 3, 'p', 4, 'q', 5, 'r', 6, 'wing_alpha', 7, 'wing_beta', 8, 'wing_RPM', 9, 'left_alpha', 10,...
    'right_alpha', 11, 'left_beta', 12, 'right_beta', 13, 'wing_prop_alpha', 14, 'wing_prop_beta', 15, 'tail_alpha', 16, 'tail_beta', 17, 'tail_RPM', 18, 'tailLeft_alpha', 19, 'tailRight_alpha', 20,...
    'tailLeft_beta', 21, 'tailRight_beta', 22, 'tail_prop_alpha', 23, 'tail_prop_beta', 24, 'Q', 25, 'aileron', 26, 'elevator', 27, 'flap', 28, 'rudder', 29, 'wing_tilt', 30,...
    'tail_tilt', 31, 'RPM_tailLeft', 32, 'RPM_tailRight', 33, 'RPM_leftOut1', 34, 'RPM_left2', 35, 'RPM_left3', 36, 'RPM_left4', 37, 'RPM_left5', 38, 'RPM_left6In', 39, 'RPM_right7In', 40,...
    'RPM_right8', 41, 'RPM_right9', 42, 'RPM_right10', 43, 'RPM_right11', 44, 'RPM_right12Out', 45);

interp_point_1  = u(variable_indices.U);
interp_point_2  = u(variable_indices.wing_RPM);
interp_point_3  = u(variable_indices.wing_prop_alpha);
interp_point_4  = u(variable_indices.wing_prop_beta);

end

% y = [U, alpha, beta, p, q, r, wing_alpha, wing_beta, wing_RPM, left_alpha, right_alpha, left_beta, right_beta, wing_prop_alpha, wing_prop_beta, ...
    % tail_alpha, tail_beta, tail_RPM, tailLeft_alpha, tailRight_alpha, tailLeft_beta, tailRight_beta, tail_prop_alpha, ...
    % tail_prop_beta, Q, aileron, elevator, flap, rudder, wing_tilt, tail_tilt, RPM_tailLeft, RPM_tailRight, RPM_leftOut1, RPM_left2, ...
    % RPM_left3, RPM_left4, RPM_left5, RPM_left6In, RPM_right7In, RPM_right8, RPM_right9, RPM_right10, RPM_right11, RPM_right12Out];

== matlab function BechamoNasaOpenModels/Mavrik v1/Mavrik Aero/Kq/Kq_left_3 ==
  data: u input size=[1 45]; interp_point_1 output; interp_point_2 output; interp_point_3 output; interp_point_4 output
function [interp_point_1, interp_point_2, interp_point_3, interp_point_4] = fcn(u)

% Find Interpolation Points
variable_indices = struct('U', 1, 'alpha', 2, 'beta', 3, 'p', 4, 'q', 5, 'r', 6, 'wing_alpha', 7, 'wing_beta', 8, 'wing_RPM', 9, 'left_alpha', 10,...
    'right_alpha', 11, 'left_beta', 12, 'right_beta', 13, 'wing_prop_alpha', 14, 'wing_prop_beta', 15, 'tail_alpha', 16, 'tail_beta', 17, 'tail_RPM', 18, 'tailLeft_alpha', 19, 'tailRight_alpha', 20,...
    'tailLeft_beta', 21, 'tailRight_beta', 22, 'tail_prop_alpha', 23, 'tail_prop_beta', 24, 'Q', 25, 'aileron', 26, 'elevator', 27, 'flap', 28, 'rudder', 29, 'wing_tilt', 30,...
    'tail_tilt', 31, 'RPM_tailLeft', 32, 'RPM_tailRight', 33, 'RPM_leftOut1', 34, 'RPM_left2', 35, 'RPM_left3', 36, 'RPM_left4', 37, 'RPM_left5', 38, 'RPM_left6In', 39, 'RPM_right7In', 40,...
    'RPM_right8', 41, 'RPM_right9', 42, 'RPM_right10', 43, 'RPM_right11', 44, 'RPM_right12Out', 45);

interp_point_1  = u(variable_indices.U);
interp_point_2  = u(variable_indices.wing_RPM);
interp_point_3  = u(variable_indices.wing_prop_alpha);
interp_point_4  = u(variable_indices.wing_prop_beta);

end

% y = [U, alpha, beta, p, q, r, wing_alpha, wing_beta, wing_RPM, left_alpha, right_alpha, left_beta, right_beta, wing_prop_alpha, wing_prop_beta, ...
    % tail_alpha, tail_beta, tail_RPM, tailLeft_alpha, tailRight_alpha, tailLeft_beta, tailRight_beta, tail_prop_alpha, ...
    % tail_prop_beta, Q, aileron, elevator, flap, rudder, wing_tilt, tail_tilt, RPM_tailLeft, RPM_tailRight, RPM_leftOut1, RPM_left2, ...
    % RPM_left3, RPM_left4, RPM_left5, RPM_left6In, RPM_right7In, RPM_right8, RPM_right9, RPM_right10, RPM_right11, RPM_right12Out];

== matlab function BechamoNasaOpenModels/Mavrik v1/Mavrik Aero/Kq/Kq_left_6_in ==
  data: u input size=[1 45]; interp_point_1 output; interp_point_2 output; interp_point_3 output; interp_point_4 output
function [interp_point_1, interp_point_2, interp_point_3, interp_point_4] = fcn(u)

% Find Interpolation Points
variable_indices = struct('U', 1, 'alpha', 2, 'beta', 3, 'p', 4, 'q', 5, 'r', 6, 'wing_alpha', 7, 'wing_beta', 8, 'wing_RPM', 9, 'left_alpha', 10,...
    'right_alpha', 11, 'left_beta', 12, 'right_beta', 13, 'wing_prop_alpha', 14, 'wing_prop_beta', 15, 'tail_alpha', 16, 'tail_beta', 17, 'tail_RPM', 18, 'tailLeft_alpha', 19, 'tailRight_alpha', 20,...
    'tailLeft_beta', 21, 'tailRight_beta', 22, 'tail_prop_alpha', 23, 'tail_prop_beta', 24, 'Q', 25, 'aileron', 26, 'elevator', 27, 'flap', 28, 'rudder', 29, 'wing_tilt', 30,...
    'tail_tilt', 31, 'RPM_tailLeft', 32, 'RPM_tailRight', 33, 'RPM_leftOut1', 34, 'RPM_left2', 35, 'RPM_left3', 36, 'RPM_left4', 37, 'RPM_left5', 38, 'RPM_left6In', 39, 'RPM_right7In', 40,...
    'RPM_right8', 41, 'RPM_right9', 42, 'RPM_right10', 43, 'RPM_right11', 44, 'RPM_right12Out', 45);

interp_point_1  = u(variable_indices.U);
interp_point_2  = u(variable_indices.wing_RPM);
interp_point_3  = u(variable_indices.wing_prop_alpha);
interp_point_4  = u(variable_indices.wing_prop_beta);

end

% y = [U, alpha, beta, p, q, r, wing_alpha, wing_beta, wing_RPM, left_alpha, right_alpha, left_beta, right_beta, wing_prop_alpha, wing_prop_beta, ...
    % tail_alpha, tail_beta, tail_RPM, tailLeft_alpha, tailRight_alpha, tailLeft_beta, tailRight_beta, tail_prop_alpha, ...
    % tail_prop_beta, Q, aileron, elevator, flap, rudder, wing_tilt, tail_tilt, RPM_tailLeft, RPM_tailRight, RPM_leftOut1, RPM_left2, ...
    % RPM_left3, RPM_left4, RPM_left5, RPM_left6In, RPM_right7In, RPM_right8, RPM_right9, RPM_right10, RPM_right11, RPM_right12Out];

== matlab function BechamoNasaOpenModels/Mavrik v1/Mavrik Aero/Kq/Kq_left_4 ==
  data: u input size=[1 45]; interp_point_1 output; interp_point_2 output; interp_point_3 output; interp_point_4 output
function [interp_point_1, interp_point_2, interp_point_3, interp_point_4] = fcn(u)

% Find Interpolation Points
variable_indices = struct('U', 1, 'alpha', 2, 'beta', 3, 'p', 4, 'q', 5, 'r', 6, 'wing_alpha', 7, 'wing_beta', 8, 'wing_RPM', 9, 'left_alpha', 10,...
    'right_alpha', 11, 'left_beta', 12, 'right_beta', 13, 'wing_prop_alpha', 14, 'wing_prop_beta', 15, 'tail_alpha', 16, 'tail_beta', 17, 'tail_RPM', 18, 'tailLeft_alpha', 19, 'tailRight_alpha', 20,...
    'tailLeft_beta', 21, 'tailRight_beta', 22, 'tail_prop_alpha', 23, 'tail_prop_beta', 24, 'Q', 25, 'aileron', 26, 'elevator', 27, 'flap', 28, 'rudder', 29, 'wing_tilt', 30,...
    'tail_tilt', 31, 'RPM_tailLeft', 32, 'RPM_tailRight', 33, 'RPM_leftOut1', 34, 'RPM_left2', 35, 'RPM_left3', 36, 'RPM_left4', 37, 'RPM_left5', 38, 'RPM_left6In', 39, 'RPM_right7In', 40,...
    'RPM_right8', 41, 'RPM_right9', 42, 'RPM_right10', 43, 'RPM_right11', 44, 'RPM_right12Out', 45);

interp_point_1  = u(variable_indices.U);
interp_point_2  = u(variable_indices.wing_RPM);
interp_point_3  = u(variable_indices.wing_prop_alpha);
interp_point_4  = u(variable_indices.wing_prop_beta);

end

% y = [U, alpha, beta, p, q, r, wing_alpha, wing_beta, wing_RPM, left_alpha, right_alpha, left_beta, right_beta, wing_prop_alpha, wing_prop_beta, ...
    % tail_alpha, tail_beta, tail_RPM, tailLeft_alpha, tailRight_alpha, tailLeft_beta, tailRight_beta, tail_prop_alpha, ...
    % tail_prop_beta, Q, aileron, elevator, flap, rudder, wing_tilt, tail_tilt, RPM_tailLeft, RPM_tailRight, RPM_leftOut1, RPM_left2, ...
    % RPM_left3, RPM_left4, RPM_left5, RPM_left6In, RPM_right7In, RPM_right8, RPM_right9, RPM_right10, RPM_right11, RPM_right12Out];

== matlab function BechamoNasaOpenModels/Mavrik v1/Mavrik Aero/Kq/Kq_left_5 ==
  data: u input size=[1 45]; interp_point_1 output; interp_point_2 output; interp_point_3 output; interp_point_4 output
function [interp_point_1, interp_point_2, interp_point_3, interp_point_4] = fcn(u)

% Find Interpolation Points
variable_indices = struct('U', 1, 'alpha', 2, 'beta', 3, 'p', 4, 'q', 5, 'r', 6, 'wing_alpha', 7, 'wing_beta', 8, 'wing_RPM', 9, 'left_alpha', 10,...
    'right_alpha', 11, 'left_beta', 12, 'right_beta', 13, 'wing_prop_alpha', 14, 'wing_prop_beta', 15, 'tail_alpha', 16, 'tail_beta', 17, 'tail_RPM', 18, 'tailLeft_alpha', 19, 'tailRight_alpha', 20,...
    'tailLeft_beta', 21, 'tailRight_beta', 22, 'tail_prop_alpha', 23, 'tail_prop_beta', 24, 'Q', 25, 'aileron', 26, 'elevator', 27, 'flap', 28, 'rudder', 29, 'wing_tilt', 30,...
    'tail_tilt', 31, 'RPM_tailLeft', 32, 'RPM_tailRight', 33, 'RPM_leftOut1', 34, 'RPM_left2', 35, 'RPM_left3', 36, 'RPM_left4', 37, 'RPM_left5', 38, 'RPM_left6In', 39, 'RPM_right7In', 40,...
    'RPM_right8', 41, 'RPM_right9', 42, 'RPM_right10', 43, 'RPM_right11', 44, 'RPM_right12Out', 45);

interp_point_1  = u(variable_indices.U);
interp_point_2  = u(variable_indices.wing_RPM);
interp_point_3  = u(variable_indices.wing_prop_alpha);
interp_point_4  = u(variable_indices.wing_prop_beta);

end

% y = [U, alpha, beta, p, q, r, wing_alpha, wing_beta, wing_RPM, left_alpha, right_alpha, left_beta, right_beta, wing_prop_alpha, wing_prop_beta, ...
    % tail_alpha, tail_beta, tail_RPM, tailLeft_alpha, tailRight_alpha, tailLeft_beta, tailRight_beta, tail_prop_alpha, ...
    % tail_prop_beta, Q, aileron, elevator, flap, rudder, wing_tilt, tail_tilt, RPM_tailLeft, RPM_tailRight, RPM_leftOut1, RPM_left2, ...
    % RPM_left3, RPM_left4, RPM_left5, RPM_left6In, RPM_right7In, RPM_right8, RPM_right9, RPM_right10, RPM_right11, RPM_right12Out];

== matlab function BechamoNasaOpenModels/Mavrik v1/Mavrik Aero/Kq/Kq_left_out ==
  data: u input size=[1 45]; interp_point_1 output; interp_point_2 output; interp_point_3 output; interp_point_4 output
function [interp_point_1, interp_point_2, interp_point_3, interp_point_4] = fcn(u)

% Find Interpolation Points
variable_indices = struct('U', 1, 'alpha', 2, 'beta', 3, 'p', 4, 'q', 5, 'r', 6, 'wing_alpha', 7, 'wing_beta', 8, 'wing_RPM', 9, 'left_alpha', 10,...
    'right_alpha', 11, 'left_beta', 12, 'right_beta', 13, 'wing_prop_alpha', 14, 'wing_prop_beta', 15, 'tail_alpha', 16, 'tail_beta', 17, 'tail_RPM', 18, 'tailLeft_alpha', 19, 'tailRight_alpha', 20,...
    'tailLeft_beta', 21, 'tailRight_beta', 22, 'tail_prop_alpha', 23, 'tail_prop_beta', 24, 'Q', 25, 'aileron', 26, 'elevator', 27, 'flap', 28, 'rudder', 29, 'wing_tilt', 30,...
    'tail_tilt', 31, 'RPM_tailLeft', 32, 'RPM_tailRight', 33, 'RPM_leftOut1', 34, 'RPM_left2', 35, 'RPM_left3', 36, 'RPM_left4', 37, 'RPM_left5', 38, 'RPM_left6In', 39, 'RPM_right7In', 40,...
    'RPM_right8', 41, 'RPM_right9', 42, 'RPM_right10', 43, 'RPM_right11', 44, 'RPM_right12Out', 45);

interp_point_1  = u(variable_indices.U);
interp_point_2  = u(variable_indices.wing_RPM);
interp_point_3  = u(variable_indices.wing_prop_alpha);
interp_point_4  = u(variable_indices.wing_prop_beta);

end

% y = [U, alpha, beta, p, q, r, wing_alpha, wing_beta, wing_RPM, left_alpha, right_alpha, left_beta, right_beta, wing_prop_alpha, wing_prop_beta, ...
    % tail_alpha, tail_beta, tail_RPM, tailLeft_alpha, tailRight_alpha, tailLeft_beta, tailRight_beta, tail_prop_alpha, ...
    % tail_prop_beta, Q, aileron, elevator, flap, rudder, wing_tilt, tail_tilt, RPM_tailLeft, RPM_tailRight, RPM_leftOut1, RPM_left2, ...
    % RPM_left3, RPM_left4, RPM_left5, RPM_left6In, RPM_right7In, RPM_right8, RPM_right9, RPM_right10, RPM_right11, RPM_right12Out];

== matlab function BechamoNasaOpenModels/Mavrik v1/Mavrik Aero/Kq/Kq_right_10 ==
  data: u input size=[1 45]; interp_point_1 output; interp_point_2 output; interp_point_3 output; interp_point_4 output
function [interp_point_1, interp_point_2, interp_point_3, interp_point_4] = fcn(u)

% Find Interpolation Points
variable_indices = struct('U', 1, 'alpha', 2, 'beta', 3, 'p', 4, 'q', 5, 'r', 6, 'wing_alpha', 7, 'wing_beta', 8, 'wing_RPM', 9, 'left_alpha', 10,...
    'right_alpha', 11, 'left_beta', 12, 'right_beta', 13, 'wing_prop_alpha', 14, 'wing_prop_beta', 15, 'tail_alpha', 16, 'tail_beta', 17, 'tail_RPM', 18, 'tailLeft_alpha', 19, 'tailRight_alpha', 20,...
    'tailLeft_beta', 21, 'tailRight_beta', 22, 'tail_prop_alpha', 23, 'tail_prop_beta', 24, 'Q', 25, 'aileron', 26, 'elevator', 27, 'flap', 28, 'rudder', 29, 'wing_tilt', 30,...
    'tail_tilt', 31, 'RPM_tailLeft', 32, 'RPM_tailRight', 33, 'RPM_leftOut1', 34, 'RPM_left2', 35, 'RPM_left3', 36, 'RPM_left4', 37, 'RPM_left5', 38, 'RPM_left6In', 39, 'RPM_right7In', 40,...
    'RPM_right8', 41, 'RPM_right9', 42, 'RPM_right10', 43, 'RPM_right11', 44, 'RPM_right12Out', 45);

interp_point_1  = u(variable_indices.U);
interp_point_2  = u(variable_indices.wing_RPM);
interp_point_3  = u(variable_indices.wing_prop_alpha);
interp_point_4  = u(variable_indices.wing_prop_beta);

end

% y = [U, alpha, beta, p, q, r, wing_alpha, wing_beta, wing_RPM, left_alpha, right_alpha, left_beta, right_beta, wing_prop_alpha, wing_prop_beta, ...
    % tail_alpha, tail_beta, tail_RPM, tailLeft_alpha, tailRight_alpha, tailLeft_beta, tailRight_beta, tail_prop_alpha, ...
    % tail_prop_beta, Q, aileron, elevator, flap, rudder, wing_tilt, tail_tilt, RPM_tailLeft, RPM_tailRight, RPM_leftOut1, RPM_left2, ...
    % RPM_left3, RPM_left4, RPM_left5, RPM_left6In, RPM_right7In, RPM_right8, RPM_right9, RPM_right10, RPM_right11, RPM_right12Out];

== matlab function BechamoNasaOpenModels/Mavrik v1/Mavrik Aero/Kq/Kq_right_12_out ==
  data: u input size=[1 45]; interp_point_1 output; interp_point_2 output; interp_point_3 output; interp_point_4 output
function [interp_point_1, interp_point_2, interp_point_3, interp_point_4] = fcn(u)

% Find Interpolation Points
variable_indices = struct('U', 1, 'alpha', 2, 'beta', 3, 'p', 4, 'q', 5, 'r', 6, 'wing_alpha', 7, 'wing_beta', 8, 'wing_RPM', 9, 'left_alpha', 10,...
    'right_alpha', 11, 'left_beta', 12, 'right_beta', 13, 'wing_prop_alpha', 14, 'wing_prop_beta', 15, 'tail_alpha', 16, 'tail_beta', 17, 'tail_RPM', 18, 'tailLeft_alpha', 19, 'tailRight_alpha', 20,...
    'tailLeft_beta', 21, 'tailRight_beta', 22, 'tail_prop_alpha', 23, 'tail_prop_beta', 24, 'Q', 25, 'aileron', 26, 'elevator', 27, 'flap', 28, 'rudder', 29, 'wing_tilt', 30,...
    'tail_tilt', 31, 'RPM_tailLeft', 32, 'RPM_tailRight', 33, 'RPM_leftOut1', 34, 'RPM_left2', 35, 'RPM_left3', 36, 'RPM_left4', 37, 'RPM_left5', 38, 'RPM_left6In', 39, 'RPM_right7In', 40,...
    'RPM_right8', 41, 'RPM_right9', 42, 'RPM_right10', 43, 'RPM_right11', 44, 'RPM_right12Out', 45);

interp_point_1  = u(variable_indices.U);
interp_point_2  = u(variable_indices.wing_RPM);
interp_point_3  = u(variable_indices.wing_prop_alpha);
interp_point_4  = u(variable_indices.wing_prop_beta);

end

% y = [U, alpha, beta, p, q, r, wing_alpha, wing_beta, wing_RPM, left_alpha, right_alpha, left_beta, right_beta, wing_prop_alpha, wing_prop_beta, ...
    % tail_alpha, tail_beta, tail_RPM, tailLeft_alpha, tailRight_alpha, tailLeft_beta, tailRight_beta, tail_prop_alpha, ...
    % tail_prop_beta, Q, aileron, elevator, flap, rudder, wing_tilt, tail_tilt, RPM_tailLeft, RPM_tailRight, RPM_leftOut1, RPM_left2, ...
    % RPM_left3, RPM_left4, RPM_left5, RPM_left6In, RPM_right7In, RPM_right8, RPM_right9, RPM_right10, RPM_right11, RPM_right12Out];

== matlab function BechamoNasaOpenModels/Mavrik v1/Mavrik Aero/Cx/CX_wing ==
  data: u input size=[1 45]; interp_point_1 output; interp_point_2 output; interp_point_3 output; interp_point_4 output; interp_point_5 output; interp_point_6 output
function [interp_point_1, interp_point_2, interp_point_3, interp_point_4, interp_point_5, interp_point_6] = fcn(u)

% Find Interpolation Points
variable_indices = struct('U', 1, 'alpha', 2, 'beta', 3, 'p', 4, 'q', 5, 'r', 6, 'wing_alpha', 7, 'wing_beta', 8, 'wing_RPM', 9, 'left_alpha', 10,...
    'right_alpha', 11, 'left_beta', 12, 'right_beta', 13, 'wing_prop_alpha', 14, 'wing_prop_beta', 15, 'tail_alpha', 16, 'tail_beta', 17, 'tail_RPM', 18, 'tailLeft_alpha', 19, 'tailRight_alpha', 20,...
    'tailLeft_beta', 21, 'tailRight_beta', 22, 'tail_prop_alpha', 23, 'tail_prop_beta', 24, 'Q', 25, 'aileron', 26, 'elevator', 27, 'flap', 28, 'rudder', 29, 'wing_tilt', 30,...
    'tail_tilt', 31, 'RPM_tailLeft', 32, 'RPM_tailRight', 33, 'RPM_leftOut1', 34, 'RPM_left2', 35, 'RPM_left3', 36, 'RPM_left4', 37, 'RPM_left5', 38, 'RPM_left6In', 39, 'RPM_right7In', 40,...
    'RPM_right8', 41, 'RPM_right9', 42, 'RPM_right10', 43, 'RPM_right11', 44, 'RPM_right12Out', 45);

interp_point_1  = u(variable_indices.wing_alpha);
interp_point_2  = u(variable_indices.wing_beta);
interp_point_3  = u(variable_indices.U);
interp_point_4  = u(variable_indices.wing_RPM);
interp_point_5  = u(variable_indices.wing_prop_alpha);
interp_point_6  = u(variable_indices.wing_prop_beta);

end

% y = [U, alpha, beta, p, q, r, wing_alpha, wing_beta, wing_RPM, left_alpha, right_alpha, left_beta, right_beta, wing_prop_alpha, wing_prop_beta, ...
    % tail_alpha, tail_beta, tail_RPM, tailLeft_alpha, tailRight_alpha, tailLeft_beta, tailRight_beta, tail_prop_alpha, ...
    % tail_prop_beta, Q, aileron, elevator, flap, rudder, wing_tilt, tail_tilt, RPM_tailLeft, RPM_tailRight, RPM_leftOut1, RPM_left2, ...
    % RPM_left3, RPM_left4, RPM_left5, RPM_left6In, RPM_right7In, RPM_right8, RPM_right9, RPM_right10, RPM_right11, RPM_right12Out];
